simulink model "sistema"  (R2025b)
settings: Solver=ode1  StartTime=0.0  StopTime=100  FixedStep=0.01  RelTol=1e-3
settings Model: Creator=BioMath  LastModifiedBy=BioMath
settings DataIOCC: ReturnWorkspaceOutputs=off  TimeSaveName=t

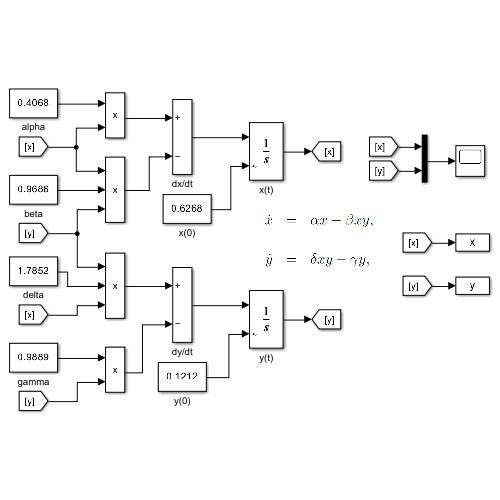
[thumbnail: Simulink's stored preview of the top-level diagram]
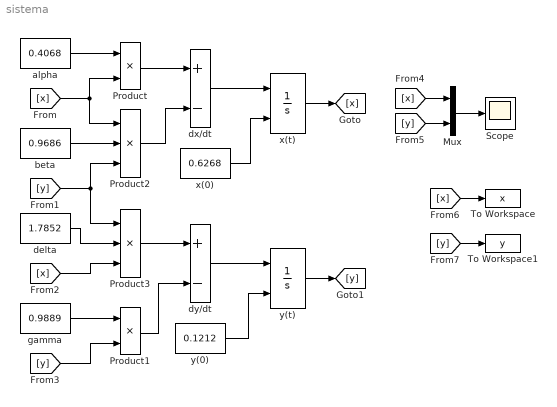
== system sistema ==
  Mux : Mux  Inputs=2
  Product : Product
  Product1 : Product
  Product2 : Product  Inputs=3
  Product3 : Product  Inputs=3
  Scope : Scope
      settings: ActiveDisplayYMinimum=-0.0653821979411443  ActiveDisplayYMaximum=1.2365659872395911
  To Workspace : ToWorkspace  VariableName=x  SampleTime=-1
  To Workspace1 : ToWorkspace  VariableName=y  SampleTime=-1
  alpha : Constant  Value=0.4068
  beta : Constant  Value=0.9686
  delta : Constant  Value=1.7852
  dx/dt : Sum  Inputs=+-
  dy/dt : Sum  Inputs=+-
  gamma : Constant  Value=0.9889
  x(0) : Constant  Value=0.6268
  x(t) : Integrator  InitialConditionSource=external
  y(0) : Constant  Value=0.1212
  y(t) : Integrator  InitialConditionSource=external
  wires:
  Product/1 -> dx/dt/1
  Product2/1 -> dx/dt/2
  x(0)/1 -> x(t)/2
  y(0)/1 -> y(t)/2
  dy/dt/1 -> y(t)/1
  dx/dt/1 -> x(t)/1
  x(t)/1 -> [x]
  y(t)/1 -> [y]
  alpha/1 -> Product/1
  [x] -> Product2/1, Product/2
  beta/1 -> Product2/2
  [y] -> Product3/1, Product2/3
  Product3/1 -> dy/dt/1
  Product1/1 -> dy/dt/2
  [x] -> Product3/3
  delta/1 -> Product3/2
  gamma/1 -> Product1/1
  [y] -> Product1/2
  Mux/1 -> Scope/1
  [x] -> Mux/1
  [y] -> Mux/2
  [x] -> To Workspace/1
  [y] -> To Workspace1/1
